simulink library "sm_stewart_platform_lib"  (R2021b)
settings: Solver=ode45  StartTime=0.0  StopTime=10.0  RelTol=1e-3  EnableMultiTasking=on
values from neighbouring files (symbols this model uses):
  s = cos(angle / 2)    [sm_stewart_platform_setup.m]
undefined symbols (not defined in the file or in its folder): hex_rad, kind_val, X, Y, Z
libraries: sm_lib x31, $bdroot x15, nesl_utility x3
(part 1 of 2)
settings Model: FPTRunName=Active  Creator=The MathWorks, Inc.  LastModifiedBy=The MathWorks, Inc.
settings SolverCC: AlgebraicLoopSolver=TrustRegion
settings DataIOCC: LimitDataPoints=on  SaveFormat=Array  SignalLoggingSaveFormat=ModelDataLogs  ReturnWorkspaceOutputs=off
settings OptimizationCC: ExpressionDepthLimit=2147483647  LifeSpan=inf
settings DebuggingCC: UnderspecifiedInitializationDetection=Classic  MergeDetectMultiDrivingBlocksExec=none  SolverPrmCheckMsg=warning  FcnCallInpInsideContextMsg=warning  StateNameClashWarn=warning  SFUnexpectedBacktrackingDiag=warning  SFNoUnconditionalDefaultTransitionDiag=warning  SFExecutionAtInitializationDiag=none  SFMachineParentedDataDiag=warning  ArithmeticOperatorsInVariantConditions=warning
settings HardwareCC: ProdBitPerPointer=32  ProdBitPerSizeT=32  ProdBitPerPtrDiffT=32  ProdLargestAtomicFloat=None  ProdIntDivRoundTo=Undefined  ProdEndianess=Unspecified  ProdWordSize=32  ProdHWDeviceType=32-bit Generic
settings ModelReferenceCC: PropagateSignalLabelsOutOfModel=off
settings SFSimCC: SimUseLocalCustomCode=off  CustomCodeUndefinedFunction=UseInterfaceOnly
settings RTWCC: RTWUseLocalCustomCode=off
settings CodeAppCC: StateflowObjectComments=on
settings GRTTargetCC: TargetLangStandard=C89/C90 (ANSI)  CombineOutputUpdateFcns=off  GRTInterface=on
settings ConfigComp: CovMetricSettings=dw  CovSaveCumulativeToWorkspaceVar=on  CovSaveSingleToWorkspaceVar=on  CovExternalEMLEnable=off

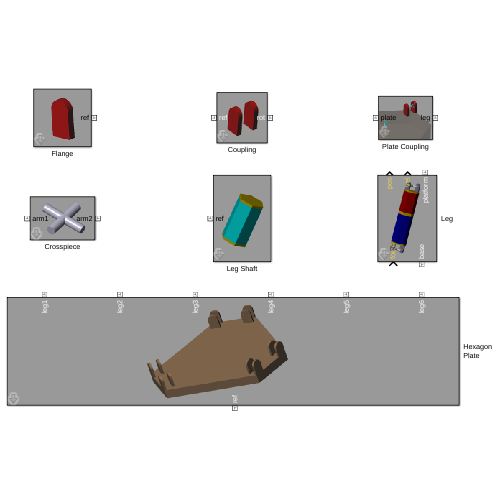
[thumbnail: Simulink's stored preview of the top-level diagram]
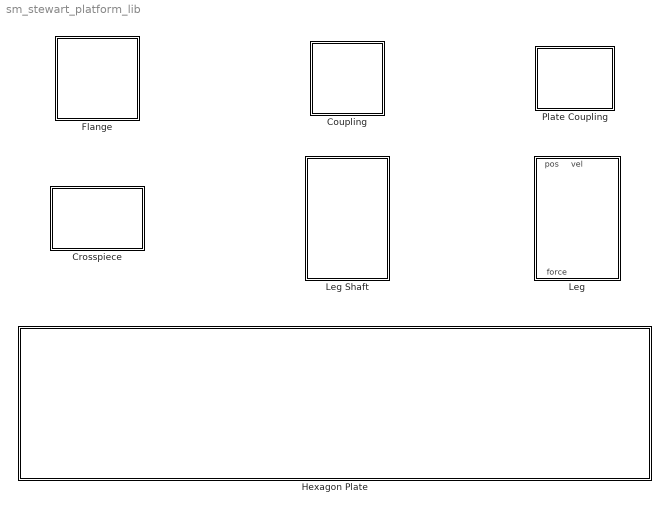
== system sm_stewart_platform_lib ==
  Coupling : Subsystem  mask(Coupling){flange_sep=2, flange_len=2, flange_width=2.25, flange_thick=0.5, ref_rot=0, diffuse=[1 0 0], specular=[0 0 0], shininess=0}
      mask prompts: flange_sep "Flange Separation (cm)"; flange_len "Flange Length (cm)"; flange_width "Flange Width (cm)"; flange_thick "Flange Thickness (cm)"; ref_rot "Reference Rotation (deg)"; diffuse "Diffuse (rgba)"; specular "Specular (rgba)"; shininess "Shininess (0-128)"
      mask help: Models a pair of parallel flanges with a revolute joint between them.
      mask Help:
      | A <em>Coupling</em> models a pair of parallel flanges with a revolute joint between them.  The axis of the revolute joint is normal to the planes of the flanges.
      | 
      | In a Stewart platform, couplings attached to the base, legs, and platform are used to anchor the arms of the universal joint crosspieces.
      | 
      | <h3>Geometry</h3>
      | 
      | The <em>Geom</em> tab parameters specify the geometry of the coupling.
      | 
      | <ul>
      | 
      | <li> <b>Flange Separation</b> The distance between the origins of the reference frames of the two flanges.  These are located within the interiors of the flanges; the distance between the facing surfaces of the flanges is one flange thickness less than this amount.
      | 
      | <li> <b>Length</b> The length of the flanges.  See <em>Flange</em> block for details.
      | 
      | <li> <b>Width</b> The width of the flanges.  See <em>Flange</em> block for details.
      | 
      | <li> <b>Thickness</b> The thickness of the flanges.  See <em>Flange</em> block for details.
      | 
      | <li> <b>Reference Rotation</b> A value specifying the zero point for the coupling's revolute joint.  A value of zero makes the zero configuration the one in which the x-axis of the <em>rot</em> frame is directed toward the curved end caps of the flanges.  A value of 180 degrees makes the zero configuration the one in which the x-axis of the <em>rot</em> frame is directed away from the curved end caps of the flanges.
      | 
      | </ul>
      | 
      | <h3>Visualization</h3>
      | 
      | The <em>Graphics</em> tab parameters specify the visualization aspects of the coupling.  Both flanges of the coupling have the same visual properties.
      | 
      | <ul>
      | 
      | <li> <b>Diffuse</b> The diffuse color of the coupling.  This is an RGB 3-vector or an RGBA 4-vector with all components in the range [0, 1].
      | 
      | <li> <b>Specular</b> The specular color of the coupling.  This is an RGB 3-vector or an RGBA 4-vector with all components in the range [0, 1].
      | 
      | <li> <b>Shininess</b> The shininess of the coupling.  This is a scalar value in the range [0, 128].
      | 
      | </ul>
      | 
      | 
      | <h3>Ports</h3>
      | 
      | <ul>
      | 
      | <li> <b>ref</b> The reference frame of the coupling.  This is also the base frame of the coupling's revolute joint.  The origin is at the midpoint of the line segment joining the reference frame origins of the two flanges.  The z-axis is normal to the planes of the flanges.  The x-axis direction depends on the setting of <em>Reference Roation</em> (see above).
      | 
      | <li> <b>rot</b> The rotated frame of the coupling.  This is also the follower frame of the coupling's revolute joint.  The origin is at the midpoint of the line segment joining the reference frame origins of the two flanges.  The z-axis is normal to the planes of the flanges.  The x-axis direction depends on the setting of <em>Reference Roation</em> (see above) and on the revolute joint's position.
      | 
      | </ul>
      | 
      | Typically, a coupling is rigidly attached to a host body through its <em>ref</em> port.  The body attached to its <em>rot</em> port can rotate about the coupling axis with respect to the host body.
      mask Display:
      | image('sm_stewart_platform_coupling.png')
      | color('white')
      | port_label('LConn', 1, 'ref')
      | port_label('RConn', 1, 'rot')
  Crosspiece : Subsystem  mask(Crosspiece){arm_len=5, arm_rad=0.5}
      mask prompts: arm_len "Arm Length (cm)"; arm_rad "Arm  Radius (cm)"
      mask help:
      | Models a solid comprising two cylinders with coincident centers and axes that intersect perpendicularly.
      |
      | A crosspieces is useful for building a detailed universal joint.  Each arm of the crosspiece is connected through a revolute joint to an adjoining solid.
      mask Help:
      | A <em>Crosspiece</em> models a solid comprising two cylinders with coincident centers and axes that intersect perpendicularly.
      | 
      | A crosspieces is useful for building a detailed universal joint.  Each arm of the crosspiece is connected through a revolute joint to an adjoining solid.
      | 
      | This block is not specific to the Stewart platform and could serve in any general library of solid shapes.
      | 
      | <h3>Parameters</h3>
      | 
      | <ul>
      | 
      | <li> <b>Arm Length</b> The common length of the two cylinders forming the arms of the crosspiece.
      | 
      | <li> <b>Arm Radius</b> The common radius of the two cylinders forming the arms of the crosspiece.
      | 
      | </ul>
      | 
      | <h3>Visualization</h3>
      | 
      | A crosspiece's material properties are set to give the crosspiece a specular, aluminum-like appearance.
      | 
      | <h3>Ports</h3>
      | 
      | <ul>
      | 
      | <li> <b>arm1</b> A frame with origin at the center of the crosspiece, z-axis aligned along the axis of the first cylinder of the crosspiece, and x-axis normal to the plane of the crosspiece.
      | 
      | <li> <b>arm2</b> A frame with origin at the center of the crosspiece, z-axis aligned along the axis of the second cylinder of the crosspiece, and x-axis normal to the plane of the crosspiece.
      | 
      | </ul>
      | 
      | The two cylinders of the crosspiece are identified such that the z-axis of the <em>arm1</em> frame crossed with the z-axis of the <em>arm2</em> frame is in the direction of the x-axes of both frames.
      | 
      | The origins of the two frames are coincident.  Connecting a body to each frame through a revolute joint effectively defines a universal joint between the two bodies.
      mask Display:
      | image('sm_stewart_platform_crosspiece.png')
      | port_label('LConn', 1, 'arm1')
      | port_label('RConn', 1, 'arm2')
  Flange : Subsystem  mask(Flange){len=10, width=10, thick=3, diffuse=[1 0 0], specular=[0 0 0], shininess=10}
      mask prompts: len "Length (cm)"; width "Width (cm)"; thick "Thickness (cm)"; diffuse "Diffuse (rgba)"; specular "Specular (rgba)"; shininess "Shininess (0-128)"
      mask help: Models a rectangular prism adjoined with a semicircular end cap.
      mask init:
      | res = 12; % Discretization level: 2n + 1 points around rounded end
      | rad = width / 2;
      | angles = (-res:1:+res) * pi/(2*res);
      | cross_sect = rad * [cos(angles); sin(angles)]';
      | if (len > 0.0)
      |     cross_sect = [cross_sect; -len, +rad; -len, -rad];
      | end
      mask Help:
      | A <em>Flange</em> models a rectangular prism adjoined with a semicircular end cap.
      | 
      | This block is not specific to the Stewart platform and could serve in any general library of solid shapes.
      | 
      | <h3>Geometry</h3>
      | 
      | The <em>Geom</em> tab parameters specify the geometry of the flange.
      | 
      | <ul>
      | 
      | <li> <b>Length</b> The length of the rectangular prism portion of the flange. This is the distance from the center of the circle defining the end cap to the flat face opposite the end cap.
      | 
      | <li> <b>Width</b> The width of the rectangular prism portion of the flange.  The radius of the circle defining the end cap is one-half of this distance. <li> <b>Thickness</b> The thickness of the flange.  Considering the flange as an extrusion of a planar shape, this is the extrusion distance.
      | 
      | </ul>
      | 
      | <h3>Visualization</h3>
      | 
      | The <em>Graphics</em> tab parameters specify the visualization aspects of the flange.
      | 
      | <ul>
      | 
      | <li> <b>Diffuse</b> The diffuse color of the flange.  This is an RGB 3-vector or an RGBA 4-vector with all components in the range [0, 1].
      | 
      | <li> <b>Specular</b> The specular color of the flange.  This is an RGB 3-vector or an RGBA 4-vector with all components in the range [0, 1].
      | 
      | <li> <b>Shininess</b> The shininess of the flange.  This is a scalar value in the range [0, 128].
      | 
      | </ul>
      | 
      | <h3>Ports</h3>
      | 
      | <ul>
      | 
      | <li> <b>ref</b> The reference frame of the flange.  The origin is at the center of the circle defining the semicircular endcaps, midway between the extruded faces.  The z-axis is in the extrusion direction, normal to the plane of the flange.  The x-axis is directed toward the end cap.
      mask Display:
      | image('sm_stewart_platform_flange.png')
      | port_label('RConn', 1, 'ref')
  Hexagon Plate : Subsystem  mask(Hexagon Plate){kind=base, hex_rad=16, hex_thick=2, hex_skew=-0.2, flange_sep=2, flange_len=2, flange_width=2.25, flange_thick=0.5, diffuse=[.8 .6 .4], specular=[.8 .6 .4], shininess=70}
      mask prompts: hex_rad "Hexagon Radius (cm)"; hex_thick "Hexagon Thickness (cm)"; hex_skew "Hexagon Skew"; flange_sep "Flange Separation (cm)"; flange_len "Flange Length (cm)"; flange_width "Flange Width (cm)"; flange_thick "Flange Thickness (cm)"; diffuse "Diffuse (rgba)"; specular "Specular (rgba)"
      mask help:
      | Models a rigid body formed by attaching six couplings to the corners of a skewed hexagon.
      |
      | There are two hexagon plates in a Stewart platform manipulator: one forming the grounded base, and the other forming the moveable platform.  Six legs connect the corresponding couplings of these two plates.  Both plates are modeled with this block.
      mask init:
      | % Set up a value equal to 0 or 1 based on whether
      | % this is the base or platform, respectively.  This value
      | % is used in the computations of certain variables and
      | % transforms that differ for the two types of hexagon plates.
      | if (kind == 1)
      |     kind_val = 0;  % Value for base
      | else
      |     kind_val = 1;  % Value for platform
      | end
      mask Help:
      | A <em>Hexagon Plate</em> models a rigid body formed by attaching six couplings to the corners of a skewed hexagon.
      | 
      | There are two hexagon plates in a Stewart platform manipulator: one forming the grounded base, and the other forming the moveable platform.  Six legs connect the corresponding couplings of these two plates.  Both plates are modeled with this block.
      | 
      | <h3>Skewed Hexagons</h3>
      | 
      | The main part of a hexagon plate is a </em>skewed hexagon</em>.  This is short hexagonal prism.  The cross section is based on a regular hexagon, but with the vertices perturbed according to the skew factor, a real value in the range (-0.5, +0.5).
      | 
      | The vertices of a skewed hexagon always lie on a circle centered at the origin. The ith vertex (i = 1, 2, ..., 6) is located at the intersection of the ray at angle theta_i with this circle, where theta_i is given by
      | 
      | theta_i = [ i - 1 + (-1)^(i - 1) s ] * pi/3  radians,
      | 
      | where s is the skew factor.  A skew factor of zero produces vertices around the circle at angles 0, pi/3, 2/3 pi, pi, 4/3 pi, 5/3 pi.  In other words, the vertices form a regular hexagon.
      | 
      | As the skew factor increase in magnitude, the hexagon vertices are shifted so that the shape becomes more and more triangular, as pairs of vertices approach each another.  Three of the sides of the hexagon grow longer as the other three grow shorter.  Regardless of the skew factor, the skewed hexagon exhibits 3-fold symmetry.  It exhibits 6-fold symmetry for a zero skew factor only.  When the skew factor is +/- 1, pairs of vertices overlap and the cross section becomes an equilateral triangle; this configuration is degenerate and not allowed.
      | 
      | A skew factor of -s produces the same shape as a skew factor of +s, except that the three side that lengthen under a skew factor of +s shrink under a skew factor of -s, and vice versa.  For a hexagonal plate, this affects the way couplings are placed on the hexagon.  If the skew factor is positive, the couplings are placed along the long sides of the hexagon; if the skew factor is negative, the couplings are placed along the short sides.
      | 
      | <h3>Geometry</h3>
      | 
      | The <em>Geom</em> tab parameters specify the geometry of the hexagon plate.
      | 
      | <ul>
      | 
      | <li> <b>Kind</b> An enumerated parameter with possible values of <em>base</em> or <em>platform</em>.  This affects some computations that are slightly different for the two types of hexagon plates in a Stewart platform.  The differences stem from two reasons.  First, the couplings appear on the top side of the base plate but on the underside of the platform plate.  Second, the couplings indices on the platform plate are offset by one (modulo 6) relative to the coupling indices on the base plate.  This causes the legs of the platform to lean in directions tangential to the edges of the base and platform plates, which adds stability to the manipulator.
      | 
      | <li> <b>Hexagon Radius</b> The radius of the circle on which the vertices of the hexagonal cross section lie.
      | 
      | <li> <b>Hexagon Thickness</b> The thickness (length) of the hexagonal prism forming the main part of the hexagon plate.
      | 
      | <li> <b>Hexagon Skew</b> The skew factor of the hexagonal cross section, in the range (-0.5, +0.5).  See <em>Skewed Hexagons</em> above for details.
      | 
      | </ul>
      | 
      | <h3>Flanges</h3>
      | 
      | The <em>Flanges</em> tab parameters specify the geometry of the flanges of the six couplings of the hexagonal plate.
      | 
      | <ul>
      | 
      | <li> <b>Flange Separation</b> The flange separation of the couplings of the hexagon plate.  See <em>Coupling</em> block for details.
      | 
      | <li> <b>Flange Length</b> The length of the coupling flanges. See <em>Coupling</em> block for details.
      | 
      | <li> <b>Flange Width</b> The width of the coupling flanges. See <em>Coupling</em> block for details.
      | 
      | <li> <b>Flange Thickness</b> The thickness of the coupling flanges. See <em>Coupling</em> block for details.
      | 
      | </ul>
      | 
      | <h3>Visualization</h3>
      | 
      | The <em>Graphics</em> tab parameters specify the visualization aspects of the hexagon plate.  The skewed hexagon and all six couplings share the same visual properties.
      | 
      | <ul>
      | 
      | <li> <b>Diffuse</b> The diffuse color of the hexagon plate.  This is an RGB 3-vector or an RGBA 4-vector with all components in the range [0, 1].
      | 
      | <li> <b>Specular</b> The specular color of the hexagon plate.  This is an RGB 3-vector or an RGBA 4-vector with all components in the range [0, 1].
      | 
      | <li> <b>Shininess</b> The shininess of the hexagon plate.  This is a scalar value in the range [0, 128].
      | 
      | </ul>
      | 
      | 
      | <h3>Ports</h3>
      | 
      | <ul>
      | 
      | <li> <b>ref</b> Reference frame of the hexagon plate.  The origin of this frame is located at the center of the skewed hexagon prism.  For a base plate, this frame is typically attached to ground or a supporting body.  For the platform plate, this frame is used to define an attachment point for a payload or end effector.
      | 
      | <li> <b>leg1, ..., leg6</b> Attachment frames for the six legs of the Stewart platform.  Each leg is attached to one of these six frames through one of its crosspieces.  When all six legs are connected to both hexagon plates in this manner, the result is a kinematically valid Stewart platform manipulator.
      | 
      | </ul>
      mask TypeOptions kind: base | platform
      mask Display:
      | image('sm_stewart_platform_hexagonplate.png')
      | color('white')
      | port_label('LConn', 1, 'ref')
      | port_label('RConn', 1, 'leg1')
      | port_label('RConn', 2, 'leg2')
      | port_label('RConn', 3, 'leg3')
      | port_label('RConn', 4, 'leg4')
      | port_label('RConn', 5, 'leg5')
      | port_label('RConn', 6, 'leg6')
  Leg : Subsystem  mask(Leg){upper_leg_len=9, lower_leg_len=12, rad=3, collar_thick=0.5, flange_len=2, flange_width=2.25, flange_thick=0.5, asm_offset=0}
      mask prompts: upper_leg_len "Upper Leg Length (cm)"; lower_leg_len "Lower Leg Length (cm)"; rad "Radius (cm)"; collar_thick "Collar Thickness (cm)"; flange_len "Flange Length (cm)"; flange_width "Flange Width (cm)"; flange_thick "Flange Thickness (cm)"; asm_offset "Assembly Offset (cm)"
      mask help:
      | Models one of the six identical legs of a Stewart platform manipulator.
      |
      | Each leg is attached to two couplings: one on the base plate of the manipulator and a corresponding one on the platform plate of the manipulator.
      mask Help:
      | A <em>Leg</em> models one of the six identical legs of a Stewart platform manipulator.
      | 
      | Each leg is attached to two couplings: one on the base plate of the manipulator
      | and a corresponding one on the platform plate of the manipulator.
      | 
      | <h3>Components</h3>
      | 
      | A leg is an articulated, non-rigid structure comprising the following parts, listed in
      | top-to-bottom order in the typical orientation of the manipulator.
      | 
      | <ul>
      | <li> Shoulder crosspiece
      | <li> Revolute joint
      | <li> Upper leg
      | <li> Cylindrical knee joint
      | <li> Lower leg
      | <li> Revolute joint
      | <li> Ankle crosspiece
      | </ul>
      | 
      | The two revolute joints adjacent to the two crosspieces each form one half of a universal joint.  The other halves are modeled by revolute joints in the couplings to which the leg is connected.  These connections between legs and couplings could also be modeled by Universal Joint blocks, however, modeling these universal joints with pairs of revolute joints allows for a more detailed model that can display the motion of the universal joint crosspieces.
      | 
      | The leg is divided into upper and lower segments connected through a cylindrical knee joint.  The main portion of each of the two leg segments is modeled as a leg shaft.  Both segments have couplings attached; the upper leg also has a cylindrical extender bar attached.
      | 
      | The revolute primitive of the knee joint is completely passive; it is not actuated.  It is also not sensed.  However, the degree of freedom provided by this primitive is necessary to allow the Stewart platform to move.
      | 
      | The prismatic primitive of the knee joint is force actuated.  The force to be applied to this primitive is provided through a Simulink signal input. This primitive is also sensed: its (linear) position and velocity are available as two Simulink signal outputs.  Typically, a control system will read the current position and velocity and use these to determine a force to be applied to the prismatic primitive of the knee joint to achieve a desired motion of the platform.
      | 
      | Under normal operation, the position of the prismatic primitive of the knee joint should lie within the range [0, L], where L is the length of the lower leg segment.  In the zero configuration of the joint, the upper leg just touches the lower leg, with no gap between them.  A negative joint position will cause the two leg segments to intersect.  Positions exceeding L will cause the extender bar to completely leave the lower leg segment.
      | 
      | <h3>Leg Geometry</h3>
      | 
      | The <em>Geom</em> tab parameters specify the geometry of the main parts of the leg.
      | 
      | <ul>
      | 
      | <li> <b>Upper Leg Length</b> The length of the upper segment of the leg, including the thicknesses of the hexagonal collars but excluding the coupling and extender bar.
      | 
      | <li> <b>Lower Leg Length</b> The length of the lower segment of the leg, including the thicknesses of the hexagonal collars but excluding the coupling.
      | 
      | <li> <b>Radius</b> The radius of the hexagonal cross section of the upper and lower leg segments.
      | 
      | <li> <b>Collar Thickness</b> The thicknesses of the hexagonal collars the upper and lower leg segments.
      | 
      | </ul>
      | 
      | <h3>Flanges</h3>
      | 
      | The <em>Flanges</em> tab parameters specify the geometry of the flanges of the
      | couplings attached to the upper and lower legs.
      | 
      | <ul>
      | 
      | <li> <b>Flange Length</b> The length of the coupling flanges. See <em>Coupling</em> block for details.
      | 
      | <li> <b>Flange Width</b> The width of the coupling flanges. See <em>Coupling</em> block for details.
      | 
      | <li> <b>Flange Thickness</b> The thickness of the coupling flanges. See <em>Coupling</em> block for details.
      | 
      | </ul>
      | 
      | <h3>Assembly</h3>
      | 
      | The <em>Assembly</em> tab parameters specify values to be used during assembly of the Stewart Platform manipulator.
      | 
      | <ul>
      | 
      | <li><b>Assembly Offset</b> The estimated position of the prismatic primitive of the knee joint in the assembled configuration of the Stewart platform manipulator.  This value is used as a suggested joint target for the primitive; it does not have to be exact, and it may not be achieved exactly. Nonetheless, reasonable guesses of this value increase the chances of successful assembly of the manipulator.
      | 
      | </ul>
      | 
      | 
      | <h3>Visualization</h3>
      | 
      | The material properties of a leg's components are all pre-defined and not configurable.
      | 
      | <h3>Ports</h3>
      | 
      | <ul>
      | 
      | <li> <b>base</b> The frame on the leg that should be attached to a coupling on the manipulator's base plate.  This frame is attached to the ankle crosspiece.
      | 
      | <li> <b>platform</b> The frame on the leg that should be attached to a coupling on the manipulator's platform plate.  This frame is attached to the shoulder crosspiece.
      | 
      | <li><b>pos</b> The linear position of the prismatic primitive of the leg's knee joint as a Simulink signal output.  This signal is typically an input to a controller.
      | 
      | <li><b>vel</b> The linear velocity of the prismatic primitive of the leg's knee joint as a Simulink signal output.  This signal is typically an input to a controller.
      | 
      | <li><b>force</b> The force (in N) to be applied to the prismatic primitive of the leg's knee joint as a Simulink signal input.  This signal is typically specified by an output of a controller.  A positive force tends to increase the primitive position.
      | 
      | </ul>
      mask Display:
      | image('sm_stewart_platform_leg.png')
      | color('white')
      | port_label('LConn', 1, 'base')
      | port_label('RConn', 1, 'platform')
      | color('yellow')
      | port_label('Input', 1, 'force')
      | port_label('Output', 1, 'pos')
      | port_label('Output', 2, 'vel')
  Leg Shaft : Subsystem  mask(Leg Shaft){length=10, rad=3, collar_thick=0.5, color=[.2 .6 .7]}
      mask prompts: length "Length (cm)"; rad "Radius (cm)"; collar_thick "Collar Thickness (cm)"; color "Color (rgba)"
      mask help: Models a hexagonal prism adjoined with hexagonal collars at each end.
      mask Help:
      | A <em>Leg Shaft</em> models a hexagonal prism adjoined with hexagonal collars at each end.
      | 
      | This block is a building block for the legs of the Stewart platform.  Each leg contains two leg shafts separated by a cylindrical joint.
      | 
      | <h3>Parameters</h3>
      | 
      | <ul>
      | 
      | <li> <b>Length</b> The length of the leg shaft, measured along its axis of symmetry.  This dimension includes the thicknesses of the end collars; the  length of the main part of the shaft is two collar thicknesses less than this value.
      | 
      | <li> <b>Radius</b> The radius of the leg shaft.  The cross-section of the leg shaft is a regular hexagon inscribed in a circle of this radius. <li> <b>Collar Thickness</b> The common thickness of the two end collars of the leg shaft.  This must not exceed one half of the length of the shaft.
      | 
      | <li> <b>Color</b> The color of the central portion of the leg shaft.  This is an RGB 3-vector or an RGBA 4-vector with all components in the range [0, 1].  The visual properties of the two collars are not configurable and designed to give the collars a brass appearance.
      | 
      | </ul>
      | 
      | 
      | <h3>Ports</h3>
      | 
      | <ul> <li> <b>ref</b> The reference frame of the leg shaft.  The origin is at the center of the shaft, and the z-axis is aligned with the axis of symmetry of the hexagonal prism.
      | 
      | 
      | </ul>
      mask Display:
      | image('sm_stewart_platform_legshaft.png')
      | port_label('LConn', 1, 'ref')
  Plate Coupling : Subsystem  mask(Plate Coupling){index=0, hex_rad=hex_rad, hex_skew=0, flange_width=2.25, flange_thick=0.5, flange_sep=2, flange_ref_rot=0}
      mask prompts: index "Index (1-6)"; hex_rad "Hexagon Radius (cm)"; hex_skew "Hexagon Skew"; flange_width "Flange Width (cm)"; flange_thick "Flange Thickness (cm)"; flange_sep "Flange Separation (cm)"; flange_ref_rot "Flange Reference Rotation (deg)"
      mask help: Models a coupling with a rigid transform that places it in a specific position and orientation relative to a hexagon plate.
      mask init:
      | % index is in the range [0, 6)
      | sgn = 2 * mod(index + 1, 2) - 1;  % Alternating: +1, -1
      | alpha = (floor((index + 1) / 2) * 120  - 30) * pi/180;
      | theta = (index + sgn * hex_skew) * pi/3;
      | offset = [hex_rad, -(flange_sep + flange_thick) / 2, -flange_width / 2 * sgn] * ...
      |     [0 -sin(theta) +cos(theta); 0 -sin(alpha) +cos(alpha); 0 -cos(alpha) -sin(alpha)];
      mask Help:
      | A <em>Plate Coupling</em> models a coupling with a rigid transform that places it in a specific position and orientation relative to a hexagon plate.
      | 
      | This block serves a specialized role in the modeling of Stewart platform manipulator.  It is used to define the six couplings attached to the lower (base) and upper (platform) hexagon plates of the manipulator.  The plate coupling's initialization function performs the math needed to compute the proper rigid transforms.
      | 
      | <h3>Index</h3>
      | 
      | The <em>Index</em> tab parameters specify the index of the plate coupling.
      | 
      | <ul>
      | 
      | <li> <b>Index</b> The index of the plate coupling, which is an integer in the range [1, 6].  This value indicates which of the six couplings of a hexagonal plate is being defined.  It determines the parameters of the internal rigid transforms that place the coupling at one of the six corners of the skewed hexagon in the proper orientation.
      | 
      | </ul>
      | 
      | <h3>Geometry</h3>
      | 
      | The <em>Geom</em> tab parameters specify the geometry of the plate coupling.
      | 
      | <ul>
      | 
      | <li> <b>Hexagon Radius</b> The radius of the hexagon plate that this plate coupling is attached to.  See <em>Hexagon Plate</em> block for details.
      | 
      | <li> <b>Hexagon Skew</b> The skew factor of the hexagon plate that this plate coupling is attached to.  See <em>Hexagon Plate</em> block for details.
      | 
      | <li> <b>Flange Width</b> The width of the coupling flanges. See <em>Coupling</em> block for details.
      | 
      | <li> <b>Flange Thickness</b> The thickness of the coupling flanges. See <em>Coupling</em> block for details.
      | 
      | <li> <b>Flange Separation</b> The flange separation of the coupling. See <em>Coupling</em> block for details.
      | 
      | <li> <b>Flange Reference Rotation</b> The reference rotation of the coupling.  This value is set to zero for plate couplings attached to the top face of the base plate of the Stewart platform and to 180 degrees for plate couplings attached to the underside of the platform plate.  This aligns the x-axes of all couplings in the upward direction in the zero configuration. See <em>Coupling</em> for details.
      | 
      | </ul>
      | 
      | <h3>Ports</h3>
      | 
      | <ul>
      | 
      | <li> <b>plate</b> The frame of the plate coupling that should be rigidly attached to a frame in the center of the hexagon plate.  The z-axis of this latter frame should be oriented normal to the plane of the plate, and the z-coordinate of its origin should be in the plane of the universal joints attached to the plate.
      | 
      | <li> <b>leg</b> The frame of the plate coupling that should be attached to a leg of the Stewart platform.  Specifically, one of the two crosspieces of the leg is attached to this frame.  The other crosspiece is attached to a corresponding coupling on the other hexagon plate of the manipulator.
      | 
      | </ul>
      mask Display:
      | image('sm_stewart_platform_platecoupling.png')
      | port_label('LConn', 1, 'plate')
      | port_label('RConn', 1, 'leg')

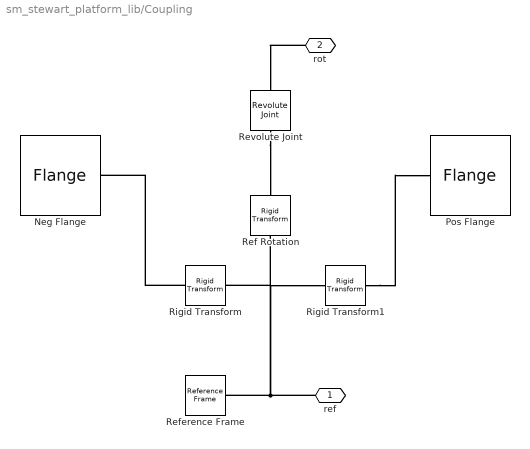
== system sm_stewart_platform_lib/Coupling ==
  Neg Flange : $bdroot/Flange  len=flange_len  width=flange_width  thick=flange_thick  diffuse=diffuse  specular=specular  shininess=shininess
  Pos Flange : $bdroot/Flange  len=flange_len  width=flange_width  thick=flange_thick  diffuse=diffuse  specular=specular  shininess=shininess
  Ref Rotation : sm_lib/Frames and Transforms/Rigid Transform  TranslationMethod=None  TranslationStandardOffset=0  TranslationLengthUnit=m  TranslationStandardAxis=+Z  TranslationCartesianOffset=[0 0 0]  TranslationROffset=0  TranslationROffsetUnits=m  TranslationZOffset=0  TranslationZOffsetUnits=m  TranslationThetaOffset=0  TranslationThetaOffsetUnits=deg  RotationMethod=StandardAxis  RotationAngleUnits=deg  RotationStandardAxis=+Z  RotationAngle=ref_rot  RotationArbitraryAxis=[0 0 1]  FollAlignAxisA=+X  BaseAlignAxisA=+Y  FollAlignAxisB=+Y  BaseAlignAxisB=+Z  RotationSequenceAxes=FollowerAxes  RotationSequence=XYX  RotationSequenceAngles=[0 0 0]  RotationSequenceAnglesUnits=deg  RotationMatrix=[1 0 0; 0 1 0; 0 0 1]
  Reference Frame : sm_lib/Frames and Transforms/Reference Frame
  Revolute Joint : sm_lib/Joints/Revolute Joint  JointMode=Normal  SenseConstraintForce=off  SenseConstraintForceX=off  SenseConstraintForceY=off  SenseConstraintForceZ=off  SenseConstraintTorque=off  SenseConstraintTorqueX=off  SenseConstraintTorqueY=off  SenseConstraintTorqueZ=off  SenseTotalForce=off  SenseTotalForceX=off  SenseTotalForceY=off  SenseTotalForceZ=off  SenseTotalTorque=off  SenseTotalTorqueX=off  SenseTotalTorqueY=off  SenseTotalTorqueZ=off  CompositeWrenchDir=FollowerOnBase  CompositeWrenchFrame=BaseFrame  EquilibriumPosition=0  EquilibriumPositionUnits=rad  SpringStiffness=0  SpringStiffnessUnits=N*m/rad  DampingCoefficient=0  DampingCoefficientUnits=N*m/(rad/s)  TorqueActuationMode=NoTorque  MotionActuationMode=ComputedMotion  SensePosition=off  SenseVelocity=off  SenseAcceleration=off  SenseTorqueForce=off  SenseLowerLimitTorqueForce=off  SenseUpperLimitTorqueForce=off  LowerLimitSpecify=off  LowerLimitBound=-90  LowerLimitBoundUnits=deg  LowerLimitStiffness=1e4  LowerLimitStiffnessUnits=N*m/deg  LowerLimitDamping=10  LowerLimitDampingUnits=N*m/(deg/s)  LowerLimitTransitionRegionWidth=0.1  LowerLimitTransitionRegionWidthUnits=deg  UpperLimitSpecify=off  UpperLimitBound=90  UpperLimitBoundUnits=deg  UpperLimitStiffness=1e4  UpperLimitStiffnessUnits=N*m/deg  UpperLimitDamping=10  UpperLimitDampingUnits=N*m/(deg/s)  UpperLimitTransitionRegionWidth=0.1  UpperLimitTransitionRegionWidthUnits=deg  PositionTargetSpecify=off  PositionTargetPriority=High  PositionTargetValue=0  PositionTargetValueUnits=rad  VelocityTargetSpecify=off  VelocityTargetPriority=High  VelocityTargetValue=0  VelocityTargetValueUnits=rad/s
  Rigid Transform : sm_lib/Frames and Transforms/Rigid Transform  TranslationMethod=StandardAxis  TranslationStandardOffset=flange_sep / 2  TranslationLengthUnit=cm  TranslationStandardAxis=-Z  TranslationCartesianOffset=[0 0 0]  TranslationROffset=0  TranslationROffsetUnits=m  TranslationZOffset=0  TranslationZOffsetUnits=m  TranslationThetaOffset=0  TranslationThetaOffsetUnits=deg  RotationMethod=None  RotationAngleUnits=deg  RotationStandardAxis=+Z  RotationAngle=0  RotationArbitraryAxis=[0 0 1]  FollAlignAxisA=+X  BaseAlignAxisA=+Y  FollAlignAxisB=+Y  BaseAlignAxisB=+Z  RotationSequenceAxes=FollowerAxes  RotationSequence=XYX  RotationSequenceAngles=[0 0 0]  RotationSequenceAnglesUnits=deg  RotationMatrix=[1 0 0; 0 1 0; 0 0 1]
  Rigid Transform1 : sm_lib/Frames and Transforms/Rigid Transform  TranslationMethod=StandardAxis  TranslationStandardOffset=flange_sep / 2  TranslationLengthUnit=cm  TranslationStandardAxis=+Z  TranslationCartesianOffset=[0 0 0]  TranslationROffset=0  TranslationROffsetUnits=m  TranslationZOffset=0  TranslationZOffsetUnits=m  TranslationThetaOffset=0  TranslationThetaOffsetUnits=deg  RotationMethod=None  RotationAngleUnits=deg  RotationStandardAxis=+Z  RotationAngle=0  RotationArbitraryAxis=[0 0 1]  FollAlignAxisA=+X  BaseAlignAxisA=+Y  FollAlignAxisB=+Y  BaseAlignAxisB=+Z  RotationSequenceAxes=FollowerAxes  RotationSequence=XYX  RotationSequenceAngles=[0 0 0]  RotationSequenceAnglesUnits=deg  RotationMatrix=[1 0 0; 0 1 0; 0 0 1]
  ref : PMIOPort  Side=Left
  rot : PMIOPort  Port=2  Side=Right
  connections:
  Rigid Transform1/LConn1 -- Rigid Transform/LConn1 -- Ref Rotation/LConn1 -- Reference Frame/RConn1 -- ref/RConn1
  Rigid Transform/RConn1 -- Neg Flange/RConn1
  Rigid Transform1/RConn1 -- Pos Flange/RConn1
  rot/RConn1 -- Revolute Joint/RConn1
  Revolute Joint/LConn1 -- Ref Rotation/RConn1

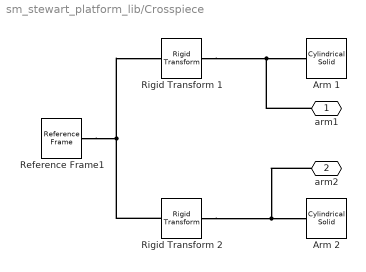
== system sm_stewart_platform_lib/Crosspiece ==
  Arm 1 : sm_lib/Body Elements/Cylindrical Solid  GraphicAmbientColor=[.9 .9 1] / 4  BasedOnType=Density  CenterOfMass=[0 0 0]  CenterOfMassUnits=m  GraphicDiffuseColor=[.9 .9 1]  CylinderLength=arm_len  CylinderLengthUnits=cm  CylinderRadius=arm_rad  CylinderRadiusUnits=cm  Density=g_density  DensityUnits=g/cm^3  DoExposeReferenceFrame=on  GraphicEmissiveColor=[0.0 0.0 0.0]  ExportEntireGeometry=off  SerializedFrames=<Frames/>  MarkerShape=Sphere  MarkerSize=1  GraphicType=FromGeometry  InertiaType=CalculateFromGeometry  Mass=1  MassUnits=kg  MomentsOfInertia=[1 1 1]  MomentsOfInertiaUnits=kg*m^2  GraphicOpacity=1  ProductsOfInertia=[0 0 0]  ProductsOfInertiaUnits=kg*m^2  GraphicShininess=100  GraphicSpecularColor=[.9 .9 1]  GraphicVisPropType=AdvancedVisualProperties
  Arm 2 : sm_lib/Body Elements/Cylindrical Solid  GraphicAmbientColor=[.9 .9 1] / 4  BasedOnType=Density  CenterOfMass=[0 0 0]  CenterOfMassUnits=m  GraphicDiffuseColor=[.9 .9 1]  CylinderLength=arm_len  CylinderLengthUnits=cm  CylinderRadius=arm_rad  CylinderRadiusUnits=cm  Density=g_density  DensityUnits=g/cm^3  DoExposeReferenceFrame=on  GraphicEmissiveColor=[0.0 0.0 0.0]  ExportEntireGeometry=off  SerializedFrames=<Frames/>  MarkerShape=Sphere  MarkerSize=1  GraphicType=FromGeometry  InertiaType=CalculateFromGeometry  Mass=1  MassUnits=kg  MomentsOfInertia=[1 1 1]  MomentsOfInertiaUnits=kg*m^2  GraphicOpacity=1  ProductsOfInertia=[0 0 0]  ProductsOfInertiaUnits=kg*m^2  GraphicShininess=100  GraphicSpecularColor=[.9 .9 1]  GraphicVisPropType=AdvancedVisualProperties
  Reference Frame1 : sm_lib/Frames and Transforms/Reference Frame
  Rigid Transform 1 : sm_lib/Frames and Transforms/Rigid Transform  TranslationMethod=None  TranslationStandardOffset=0  TranslationLengthUnit=m  TranslationStandardAxis=+Z  TranslationCartesianOffset=[0 0 0]  TranslationROffset=0  TranslationROffsetUnits=m  TranslationZOffset=0  TranslationZOffsetUnits=m  TranslationThetaOffset=0  TranslationThetaOffsetUnits=deg  RotationMethod=AlignedAxes  RotationAngleUnits=deg  RotationStandardAxis=+Z  RotationAngle=0  RotationArbitraryAxis=[0 0 1]  FollAlignAxisA=+Z  BaseAlignAxisA=+X  FollAlignAxisB=+X  BaseAlignAxisB=+Z  RotationSequenceAxes=FollowerAxes  RotationSequence=XYX  RotationSequenceAngles=[0 0 0]  RotationSequenceAnglesUnits=deg  RotationMatrix=[1 0 0; 0 1 0; 0 0 1]
  Rigid Transform 2 : sm_lib/Frames and Transforms/Rigid Transform  TranslationMethod=None  TranslationStandardOffset=0  TranslationLengthUnit=m  TranslationStandardAxis=+Z  TranslationCartesianOffset=[0 0 0]  TranslationROffset=0  TranslationROffsetUnits=m  TranslationZOffset=0  TranslationZOffsetUnits=m  TranslationThetaOffset=0  TranslationThetaOffsetUnits=deg  RotationMethod=AlignedAxes  RotationAngleUnits=deg  RotationStandardAxis=+Z  RotationAngle=0  RotationArbitraryAxis=[0 0 1]  FollAlignAxisA=+Z  BaseAlignAxisA=+Y  FollAlignAxisB=+X  BaseAlignAxisB=+Z  RotationSequenceAxes=FollowerAxes  RotationSequence=XYX  RotationSequenceAngles=[0 0 0]  RotationSequenceAnglesUnits=deg  RotationMatrix=[1 0 0; 0 1 0; 0 0 1]
  arm1 : PMIOPort  Side=Left
  arm2 : PMIOPort  Port=2  Side=Right
  connections:
  Rigid Transform 2/LConn1 -- Rigid Transform 1/LConn1 -- Reference Frame1/RConn1
  Rigid Transform 1/RConn1 -- Arm 1/RConn1 -- arm1/RConn1
  Rigid Transform 2/RConn1 -- Arm 2/RConn1 -- arm2/RConn1

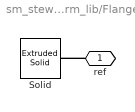
== system sm_stewart_platform_lib/Flange ==
  Solid : sm_lib/Body Elements/Extruded Solid  GraphicAmbientColor=0.1 * [1 1 1]  BasedOnType=Density  CenterOfMass=[0 0 0]  CenterOfMassUnits=m  GraphicDiffuseColor=diffuse  ExportConvexHullGeometry=off  ExtrusionCrossSection=cross_sect  ExtrusionCrossSectionUnits=cm  Density=g_density  DensityUnits=g/cm^3  DoExposeReferenceFrame=on  GraphicEmissiveColor=[0.0 0.0 0.0]  ExportEntireGeometry=off  ExtrusionLength=thick  ExtrusionLengthUnits=cm  ExtrusionType=General  SerializedFrames=<Frames/>  MarkerShape=Sphere  MarkerSize=1  GraphicType=FromGeometry  InertiaType=CalculateFromGeometry  Mass=1  MassUnits=kg  MomentsOfInertia=[1 1 1]  MomentsOfInertiaUnits=kg*m^2  PolygonNumSides=1  GraphicOpacity=1  PolygonOuterRadius=1  PolygonOuterRadiusUnits=m  ProductsOfInertia=[0 0 0]  ProductsOfInertiaUnits=kg*m^2  GraphicShininess=shininess  GraphicSpecularColor=specular  GraphicVisPropType=AdvancedVisualProperties
  ref : PMIOPort  Side=Right
  connections:
  ref/RConn1 -- Solid/RConn1

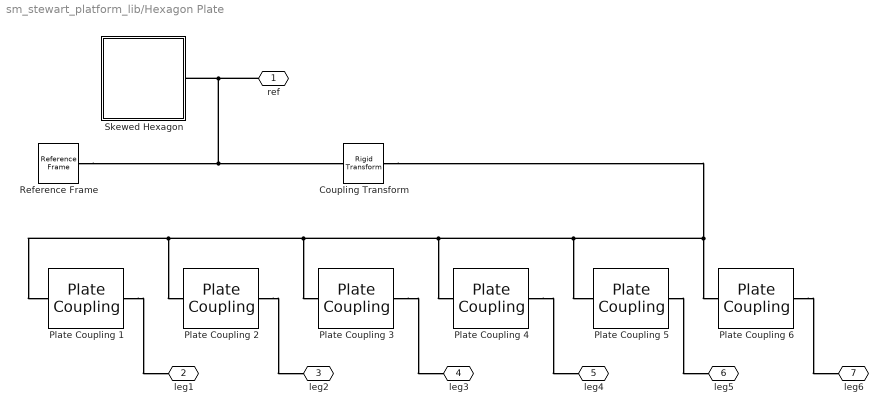
== system sm_stewart_platform_lib/Hexagon Plate ==
  Coupling Transform : sm_lib/Frames and Transforms/Rigid Transform  TranslationMethod=StandardAxis  TranslationStandardOffset=(1 - 2 * kind_val) * (hex_thick / 2 + flange_len)  TranslationLengthUnit=cm  TranslationStandardAxis=+Z  TranslationCartesianOffset=[0 0 0]  TranslationROffset=0  TranslationROffsetUnits=m  TranslationZOffset=0  TranslationZOffsetUnits=m  TranslationThetaOffset=0  TranslationThetaOffsetUnits=deg  RotationMethod=AlignedAxes  RotationAngleUnits=deg  RotationStandardAxis=+Z  RotationAngle=0  RotationArbitraryAxis=[0 0 1]  FollAlignAxisA=+Z  BaseAlignAxisA=+X  FollAlignAxisB=+X  BaseAlignAxisB=+Z  RotationSequenceAxes=FollowerAxes  RotationSequence=XYX  RotationSequenceAngles=[0 0 0]  RotationSequenceAnglesUnits=deg  RotationMatrix=[1 0 0; 0 1 0; 0 0 1]
  Plate Coupling 1 : $bdroot/Plate Coupling  index=0 + kind_val  hex_rad=hex_rad  hex_skew=hex_skew  flange_width=flange_width  flange_thick=flange_thick  flange_sep=flange_sep  flange_ref_rot=kind_val * 180
  Plate Coupling 2 : $bdroot/Plate Coupling  index=1 + kind_val  hex_rad=hex_rad  hex_skew=hex_skew  flange_width=flange_width  flange_thick=flange_thick  flange_sep=flange_sep  flange_ref_rot=kind_val * 180
  Plate Coupling 3 : $bdroot/Plate Coupling  index=2 + kind_val  hex_rad=hex_rad  hex_skew=hex_skew  flange_width=flange_width  flange_thick=flange_thick  flange_sep=flange_sep  flange_ref_rot=kind_val * 180
  Plate Coupling 4 : $bdroot/Plate Coupling  index=3 + kind_val  hex_rad=hex_rad  hex_skew=hex_skew  flange_width=flange_width  flange_thick=flange_thick  flange_sep=flange_sep  flange_ref_rot=kind_val * 180
  Plate Coupling 5 : $bdroot/Plate Coupling  index=4 + kind_val  hex_rad=hex_rad  hex_skew=hex_skew  flange_width=flange_width  flange_thick=flange_thick  flange_sep=flange_sep  flange_ref_rot=kind_val * 180
  Plate Coupling 6 : $bdroot/Plate Coupling  index=mod(5 + kind_val, 6)  hex_rad=hex_rad  hex_skew=hex_skew  flange_width=flange_width  flange_thick=flange_thick  flange_sep=flange_sep  flange_ref_rot=kind_val * 180
  Reference Frame : sm_lib/Frames and Transforms/Reference Frame
  Skewed Hexagon : Subsystem  mask(Skewed Hexagon){rad=hex_rad, thick=hex_thick, skew=hex_skew, diffuse=diffuse, specualr=specular, shininess=shininess}
      mask prompts: rad "Radius (cm)"; thick "Thickness (cm)"; diffuse "Diffuse (rgba)"; specualr "Specular (rgba)"; shininess "Shininess (0-128)"
      mask help:
      | Models a hexagonal prism with 3-fold symmetry.
      |
      | A skew factor in the range (-0.5, +0.5) controls the shape of the hexagon.  A zero skew factor produces a regular hexagon cross section, and values toward +/- 0.5 produce progressively more triangular hexagons.
      mask init:
      | angles = pi/3 * ((0:1:5) + skew * [+1 -1 +1 -1 +1 -1]);
      | cross_sect = rad * [cos(angles); sin(angles)]';
      mask Help:
      | A <em>Skewed Hexagon</em> models a hexagonal prism with 3-fold symmetry.
      | 
      | A skew factor in the range (-0.5, +0.5) controls the shape of the hexagon.  A zero
      | skew factor produces a regular hexagon cross section, and values toward +/- 0.5
      | produce progressively more triangular hexagons.
      | 
      | See <em>Skewed Hexagons</em> in the documentation of the <em>Hexagon Plate</em>
      | block for more details.
      | 
      | <h3>Geometry</h3>
      | 
      | The <em>Geom</em> tab parameters specify the geometry of the skewed hexagon.
      | 
      | <ul>
      | 
      | <li> <b>Radius</b> The radius of thee circle on which the vertices of
      |   the hexagonal cross section lie.
      | 
      | <li> <b> Thickness</b> The thickness (length) of the hexagonal prism.
      | 
      | <li> <b>Skew</b> The skew factor of the hexagonal cross section, in the
      |   range (-0.5, +0.5).
      | 
      | </ul>
      | 
      | <h3>Visualization</h3>
      | 
      | The <em>Graphics</em> tab parameters specify the visualization aspects of the skewed
      | hexagon.
      | 
      | 
      | <ul>
      | 
      | <li> <b>Diffuse</b> The diffuse color of the skewed hexagon.  This is an RGB
      | 3-vector or an RGBA 4-vector with all components in the range [0, 1].
      | 
      | <li> <b>Specular</b> The specular color of the skewed hexagon.  This is an RGB
      | 3-vector or an RGBA 4-vector with all components in the range [0, 1].
      | 
      | <li> <b>Shininess</b> The shininess of the skewed hexagon.  This is a scalar
      | value in the range [0, 128].
      | 
      | </ul>
      | 
      | 
      | <h3>Ports</h3>
      | 
      | <ul>
      | 
      | <li> <b>ref</b> Reference frame of the skewed hexagon.  The origin of this frame
      |   is located at the center of the hexagonal prism, and the z-axis is aligned
      |   with the axis of the prism.
      | 
      | </ul>
      mask Display:
      | image('sm_stewart_platform_skewedhexagon.png')
      | color('white')
      | port_label('RConn', 1, 'ref')
  ref : PMIOPort  Side=Left
  leg1 : PMIOPort  Port=2  Side=Right
  leg2 : PMIOPort  Port=3  Side=Right
  leg3 : PMIOPort  Port=4  Side=Right
  leg4 : PMIOPort  Port=5  Side=Right
  leg5 : PMIOPort  Port=6  Side=Right
  leg6 : PMIOPort  Port=7  Side=Right
  connections:
  Reference Frame/RConn1 -- ref/RConn1 -- Skewed Hexagon/RConn1 -- Coupling Transform/LConn1
  Plate Coupling 6/LConn1 -- Coupling Transform/RConn1 -- Plate Coupling 2/LConn1 -- Plate Coupling 1/LConn1 -- Plate Coupling 3/LConn1 -- Plate Coupling 4/LConn1 -- Plate Coupling 5/LConn1
  Plate Coupling 1/RConn1 -- leg1/RConn1
  Plate Coupling 2/RConn1 -- leg2/RConn1
  Plate Coupling 3/RConn1 -- leg3/RConn1
  Plate Coupling 4/RConn1 -- leg4/RConn1
  Plate Coupling 5/RConn1 -- leg5/RConn1
  Plate Coupling 6/RConn1 -- leg6/RConn1
